simulink model "lc_template"  (R2014a)
settings: Solver=FixedStepDiscrete  StartTime=0.0  StopTime=inf  FixedStep=SampleTime  RelTol=1e-3
libraries: visionstatistics x1, dspbuff3 x1, dspstat3 x1, dspmtrx3 x1
settings Model: Creator=georg  LastModifiedBy=georg

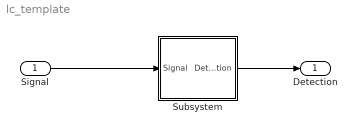
== system lc_template ==
  Signal : Inport
  Subsystem : Subsystem
  Detection : Outport
  wires:
  Signal/1 -> Subsystem/1(Signal)
  Subsystem/1(Detection) -> Detection/1

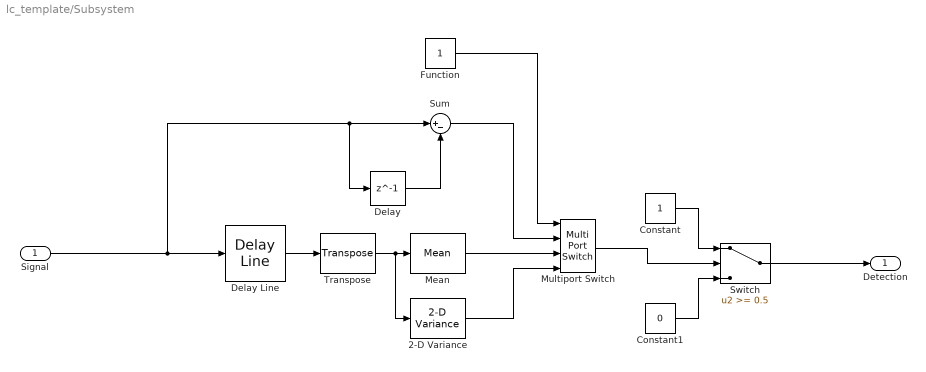
== system lc_template/Subsystem ==
  Signal : Inport
  2-D Variance : visionstatistics/2-D Variance  run=off  reset_popup=None  directionMode=Entire input  dimension=1  treatSBRowAsCol=on  roiEnable=off  roiType=Rectangles  roiPortion=Entire ROI  roiOutput=Individual statistics for each ROI  roiFlag=off  prodOutputMode=Binary point scaling  prodOutputWordLength=32  prodOutputFracLength=0  roundingMode=Floor  overflowMode=off
  Constant : Constant
  Constant1 : Constant  Value=0
  Delay : Delay  DelayLength=1  InitialCondition=0
  Delay Line : dspbuff3/Delay Line  siz=5  ic=0  directfeed=off  enable_output=off  hold_output=off  TreatMby1Signals=One channel
  Function : Constant
  Mean : dspstat3/Mean  run=off  reset_popup=None  InputProcessing=Columns as channels (frame based)  directionMode=Each column  dimension=1  treatSBRowAsCol=on  roiEnable=off  roiType=Rectangles  roiPortion=Entire ROI  roiOutput=Individual statistics for each ROI  roiFlag=off  outputDataTypeStr=Inherit: Same as accumulator  outputLastDataTypeStr=Inherit: Same as accumulator  outputMin=[]  outputMax=[]  roundingMode=Floor  overflowMode=off
  Multiport Switch : MultiPortSwitch
  Sum : Sum  Inputs=|+-
  Switch : Switch  Threshold=0.5
  Transpose : dspmtrx3/Transpose  Hermitian=off  overflowFlag=off
  Detection : Outport
  wires:
  Delay Line/1 -> Transpose/1
  Function/1 -> Multiport Switch/1
  Constant/1 -> Switch/1
  Constant1/1 -> Switch/3
  Mean/1 -> Multiport Switch/3
  Signal/1 -> Delay/1, Sum/1, Delay Line/1
  2-D Variance/1 -> Multiport Switch/4
  Switch/1 -> Detection/1
  Transpose/1 -> Mean/1, 2-D Variance/1
  Delay/1 -> Sum/2
  Multiport Switch/1 -> Switch/2
  Sum/1 -> Multiport Switch/2
